simulink model "Task2Simulink"  (R2022a)
settings: Solver=VariableStepAuto  StartTime=0.0  StopTime=10.0  RelTol=1e-3
settings Model: Creator=ahmed  LastModifiedBy=ahmed

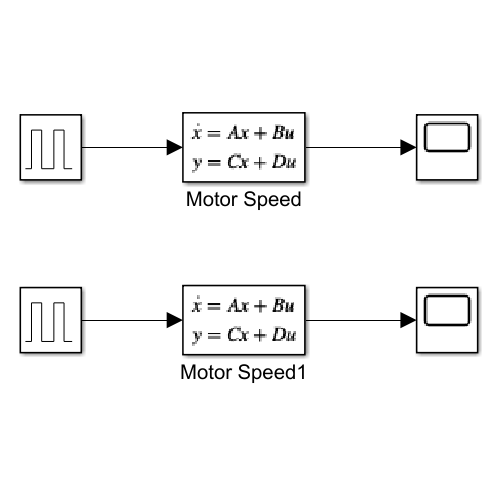
[thumbnail: Simulink's stored preview of the top-level diagram]
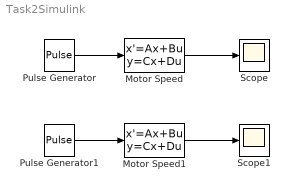
== system Task2Simulink ==
  Motor Speed : StateSpace  A="[-1.193e+04       1.951       113.2           0; 64           0           0           0;  0         128           0           0; 0           0           1           0]"  B=[64;0;0;0]  C="[ 68.56          0  -0.001724          0]"  D=0  InitialCondition=0
  Motor Speed1 : StateSpace  A="[-1.193e+04       1.951       113.2           0; 64           0           0           0;  0         128           0           0; 0           0           1           0]"  B=[64;0;0;0]  C="[ 68.56          0  -0.001724          0]"  D=0  InitialCondition=0
  Pulse Generator : DiscretePulseGenerator  PulseType=Time based  Period=10  PulseWidth=5
  Pulse Generator1 : DiscretePulseGenerator  PulseType=Time based  Period=10  PulseWidth=5
  Scope : Scope
  Scope1 : Scope
  wires:
  Motor Speed/1 -> Scope/1
  Pulse Generator/1 -> Motor Speed/1
  Motor Speed1/1 -> Scope1/1
  Pulse Generator1/1 -> Motor Speed1/1
